simulink model "Parallel4"  (Simulink 5.0)
settings: Solver=ode45  StartTime=0.0  StopTime=10.0  RelTol=1e-3
settings Model: Creator=scaife  LastModifiedBy=scaife  ExtModeAutoUpdateStatusClock=off

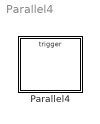
== system Parallel4 ==
  Parallel4 : Stateflow chart

== stateflow chart Parallel4 ==
  state N1/ [parallel]
    state A/
    state B/
    (default) -> A
    A -> B : S1
    B -> A : R1
  state N2/ [parallel]
    state C/
    state D/
    (default) -> C
    C -> D : S2
    D -> C : R2
  events: S1 input EITHER_EDGE_EVENT; R1 input EITHER_EDGE_EVENT; S2 input EITHER_EDGE_EVENT; R2 input EITHER_EDGE_EVENT
